simulink model "Analisis_de_Ganancias"  (R2023a)
settings: Solver=VariableStepAuto  StartTime=0.0  StopTime=10.0  RelTol=1e-3
undefined symbols (not defined in the file): alfa_inicial, area_mem, c, d, delta_f, fs, k, m, perm, Q, r1, r_ambiente1, r_ambiente2, rho, v_sonido, vel_caminata, ventana_fft, ventana_fft_analisis, zoh_freq
libraries: matrix_library x4, dspxfrm3 x2, dspvision x2, dspsnks4 x1
settings Model: Creator=tobip  LastModifiedBy=tobip

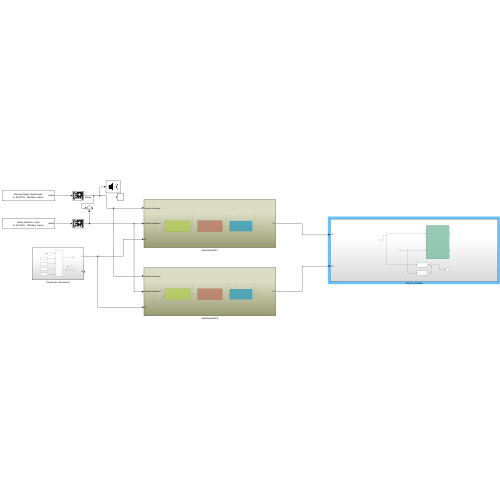
[thumbnail: Simulink's stored preview of the top-level diagram]
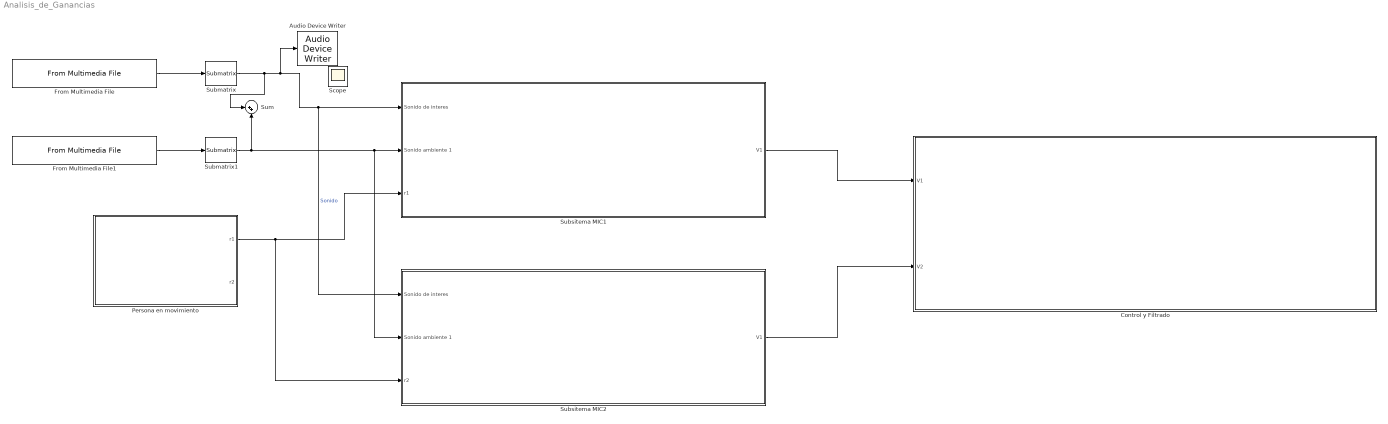
== system Analisis_de_Ganancias ==
  Audio Device Writer : dspsnks4/Audio Device Writer  Driver=DirectSound  Device=Default  InheritSampleRate=on  SampleRate=44100  BitDepth=16-bit integer  BufferSize=4096  NumBuffers=10  DefaultOutputChannelMapping=on  OutputChannelMapping=1:2  OutputNumUnderrunSamples=off  DriverIdx=1  DeviceWarnFlag=''
  Control y Filtrado : Subsystem
  From Multimedia File : dspvision/From Multimedia File  inputFilename=C:\Users\tobip\Documents\Control\Proyecto final\Audios dato\Discurso Roger Federer.mp3  readRange=[1 Inf]  loop=on  numPlays=1  outputStreams=Audio only  videoDataType=single  audioDataType=double  inheritSampleTime=on  userDefinedSampleTime=1/30  noAudioOutput=off  isIntensityVideo=off  fourcc=RGB  colorVideoFormat=Separate color signals  outputEOF=off  dataOrg=Column-major  audioFrameSize=1  computeAudioFrameSize=off  outSamplingMode=Sample based
      settings: LibrarySourceBlock=audiosources/From Multimedia File
  From Multimedia File1 : dspvision/From Multimedia File  inputFilename=C:\Users\tobip\Documents\Control\Proyecto final\Audios dato\Ruido ambiente 1.mp3  readRange=[1 Inf]  loop=on  numPlays=1  outputStreams=Audio only  videoDataType=single  audioDataType=double  inheritSampleTime=on  userDefinedSampleTime=1/30  noAudioOutput=off  isIntensityVideo=off  fourcc=RGB  colorVideoFormat=Separate color signals  outputEOF=off  dataOrg=Column-major  audioFrameSize=1  computeAudioFrameSize=off  outSamplingMode=Sample based
      settings: LibrarySourceBlock=audiosources/From Multimedia File
  Persona en movimiento : Subsystem
  Scope : Scope
  Submatrix : matrix_library/Submatrix  RowSpan=All rows  RowStartMode=First  RowStartIndex=1  RowEndMode=Middle  RowEndIndex=1  ColSpan=One column  ColStartMode=First  ColStartIndex=1  ColEndMode=Last  ColEndIndex=1
  Submatrix1 : matrix_library/Submatrix  RowSpan=All rows  RowStartMode=First  RowStartIndex=1  RowEndMode=Last  RowEndIndex=1  ColSpan=One column  ColStartMode=First  ColStartIndex=1  ColEndMode=Last  ColEndIndex=1
  Subsitema MIC1 : Subsystem
  Subsitema MIC2 : Subsystem
  Sum : Sum  Inputs=|++
  wires:
  Subsitema MIC2/1(V1) -> Control y Filtrado/2(V2)
  Persona en movimiento/1(r1) -> Subsitema MIC2/3(r2), Subsitema MIC1/3(r1)
  Submatrix1/1 -> Subsitema MIC2/2(Sonido ambiente 1), Subsitema MIC1/2(Sonido ambiente 1), Sum/2
  Submatrix/1 -> Sum/1, Audio Device Writer/1, Subsitema MIC1/1(Sonido de interes), Subsitema MIC2/1(Sonido de interes)  "Sonido"
  Subsitema MIC1/1(V1) -> Control y Filtrado/1(V1)
  From Multimedia File1/1 -> Submatrix1/1
  From Multimedia File/1 -> Submatrix/1

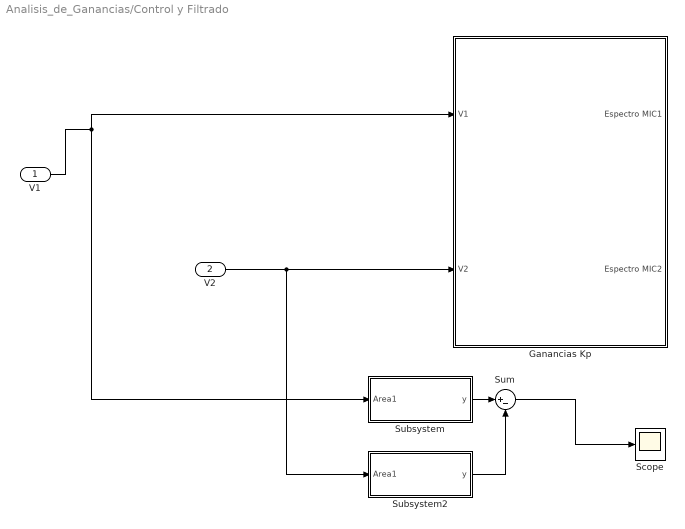
== system Analisis_de_Ganancias/Control y Filtrado ==
  V1 : Inport
  V2 : Inport  Port=2
  Ganancias Kp : Subsystem
  Scope : Scope
  Subsystem : Subsystem
  Subsystem2 : Subsystem
  Sum : Sum  Inputs=|+-
  wires:
  Subsystem/1(y) -> Sum/1
  Subsystem2/1(y) -> Sum/2
  Sum/1 -> Scope/1
  V1/1 -> Ganancias Kp/1(V1), Subsystem/1(Area1)
  V2/1 -> Ganancias Kp/2(V2), Subsystem2/1(Area1)

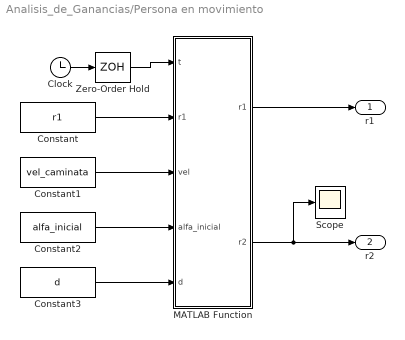
== system Analisis_de_Ganancias/Persona en movimiento ==
  Clock : Clock
  Constant : Constant  Value=r1
  Constant1 : Constant  Value=vel_caminata
  Constant2 : Constant  Value=alfa_inicial
  Constant3 : Constant  Value=d
  MATLAB Function : MATLAB Function  TreatAsAtomicUnit=on
  Scope : Scope
  Zero-Order Hold : ZeroOrderHold  SampleTime=0.1
  r1 : Outport
  r2 : Outport  Port=2
  wires:
  Constant/1 -> MATLAB Function/2("r1 ")
  Constant3/1 -> MATLAB Function/5(d)
  Constant2/1 -> MATLAB Function/4(alfa_inicial)
  Constant1/1 -> MATLAB Function/3(vel)
  Clock/1 -> Zero-Order Hold/1
  MATLAB Function/1(r1) -> r1/1
  Zero-Order Hold/1 -> MATLAB Function/1(t)
  MATLAB Function/2(r2) -> Scope/1, r2/1

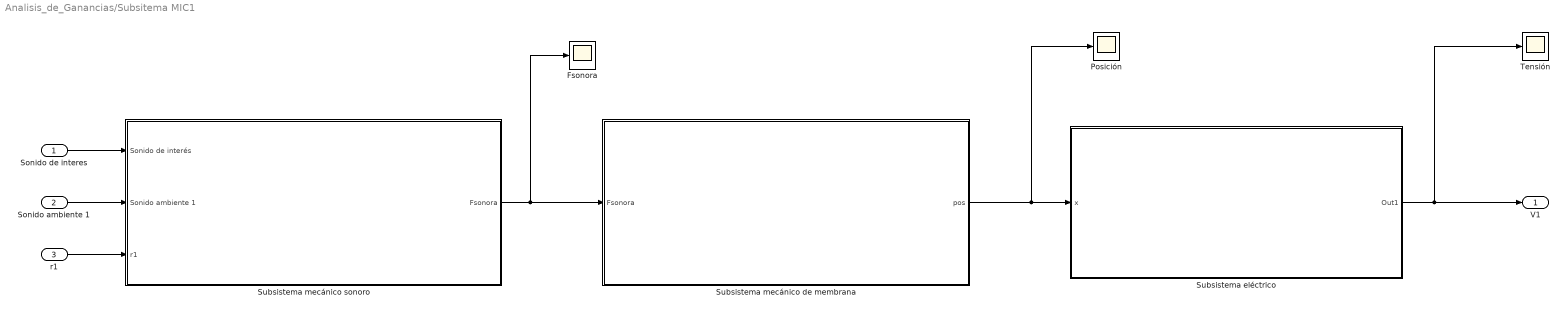
== system Analisis_de_Ganancias/Subsitema MIC1 ==
  Sonido de interes : Inport
  Sonido ambiente 1 : Inport  Port=2
  r1 : Inport  Port=3
  Fsonora : Scope
  Posición : Scope
  Subsistema eléctrico : Subsystem
  Subsistema mecánico de membrana : Subsystem
  Subsistema mecánico sonoro : Subsystem
  Tensión : Scope
  V1 : Outport
  wires:
  Subsistema mecánico de membrana/1(pos) -> Posición/1, Subsistema eléctrico/1(x)
  Sonido de interes/1 -> Subsistema mecánico sonoro/1(Sonido de interés)
  Subsistema eléctrico/1(Out1) -> Tensión/1, V1/1
  Subsistema mecánico sonoro/1(Fsonora) -> Fsonora/1, Subsistema mecánico de membrana/1(Fsonora)
  Sonido ambiente 1/1 -> Subsistema mecánico sonoro/2(Sonido ambiente 1)
  r1/1 -> Subsistema mecánico sonoro/3(r1)

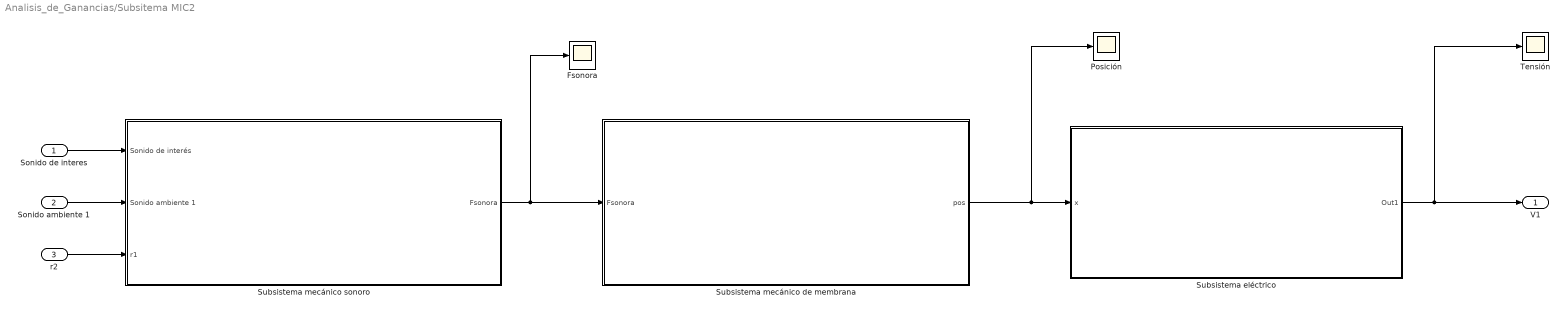
== system Analisis_de_Ganancias/Subsitema MIC2 ==
  Sonido de interes : Inport
  Sonido ambiente 1 : Inport  Port=2
  r2 : Inport  Port=3
  Fsonora : Scope
  Posición : Scope
  Subsistema eléctrico : Subsystem
  Subsistema mecánico de membrana : Subsystem
  Subsistema mecánico sonoro : Subsystem
  Tensión : Scope
  V1 : Outport
  wires:
  Subsistema mecánico de membrana/1(pos) -> Posición/1, Subsistema eléctrico/1(x)
  Sonido de interes/1 -> Subsistema mecánico sonoro/1(Sonido de interés)
  Subsistema eléctrico/1(Out1) -> Tensión/1, V1/1
  Subsistema mecánico sonoro/1(Fsonora) -> Fsonora/1, Subsistema mecánico de membrana/1(Fsonora)
  Sonido ambiente 1/1 -> Subsistema mecánico sonoro/2(Sonido ambiente 1)
  r2/1 -> Subsistema mecánico sonoro/3(r1)

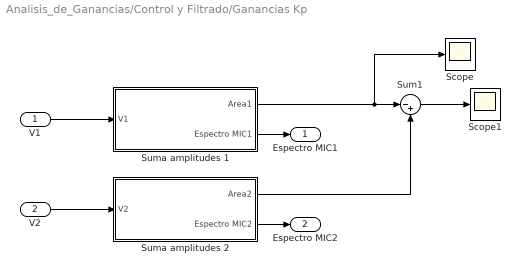
== system Analisis_de_Ganancias/Control y Filtrado/Ganancias Kp ==
  V1 : Inport
  V2 : Inport  Port=2
  Scope : Scope
  Scope1 : Scope
  Sum1 : Sum  Inputs=|-+
  Suma amplitudes 1 : Subsystem
  Suma amplitudes 2 : Subsystem
  Espectro MIC1 : Outport
  Espectro MIC2 : Outport  Port=2
  wires:
  V1/1 -> Suma amplitudes 1/1(V1)
  V2/1 -> Suma amplitudes 2/1(V2)
  Suma amplitudes 1/2(Espectro MIC1) -> Espectro MIC1/1
  Suma amplitudes 2/2(Espectro MIC2) -> Espectro MIC2/1
  Suma amplitudes 1/1(Area1) -> Scope/1, Sum1/1
  Sum1/1 -> Scope1/1
  Suma amplitudes 2/1(Area2) -> Sum1/2

== system Analisis_de_Ganancias/Control y Filtrado/Subsystem ==
  Area1 : Inport
  Buffer : Buffer  N=3  OutputFrames=off
  MATLAB Function : MATLAB Function  TreatAsAtomicUnit=on
  Zero-Order Hold : ZeroOrderHold  SampleTime=1/fs
  y : Outport
  wires:
  Buffer/1 -> MATLAB Function/1(u)
  Area1/1 -> Zero-Order Hold/1
  MATLAB Function/1(y) -> y/1
  Zero-Order Hold/1 -> Buffer/1

== system Analisis_de_Ganancias/Control y Filtrado/Subsystem2 ==
  Area1 : Inport
  Buffer : Buffer  N=3  OutputFrames=off
  MATLAB Function : MATLAB Function  TreatAsAtomicUnit=on
  Zero-Order Hold : ZeroOrderHold  SampleTime=1/fs
  y : Outport
  wires:
  Buffer/1 -> MATLAB Function/1(u)
  Area1/1 -> Zero-Order Hold/1
  MATLAB Function/1(y) -> y/1
  Zero-Order Hold/1 -> Buffer/1

== system Analisis_de_Ganancias/Subsitema MIC1/Subsistema eléctrico ==
  x : Inport
  Constant : Constant  Value=area_mem*perm
  Constant1 : Constant  Value=Q
  Divide : Product  Inputs=*/
  Divide1 : Product  Inputs=*/
  Out1 : Outport
  wires:
  x/1 -> Divide/2
  Constant/1 -> Divide/1
  Divide/1 -> Divide1/2  "Capacitancia"
  Divide1/1 -> Out1/1
  Constant1/1 -> Divide1/1

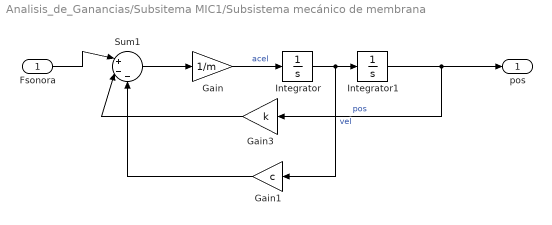
== system Analisis_de_Ganancias/Subsitema MIC1/Subsistema mecánico de membrana ==
  Fsonora : Inport
  Gain : Gain  Gain=1/m
  Gain1 : Gain  Gain=c
  Gain3 : Gain  Gain=k
  Integrator : Integrator
  Integrator1 : Integrator
  Sum1 : Sum  Inputs=|+--
  pos : Outport
  wires:
  Integrator1/1 -> Gain3/1, pos/1  "pos"
  Integrator/1 -> Gain1/1, Integrator1/1  "vel"
  Fsonora/1 -> Sum1/1
  Gain3/1 -> Sum1/2
  Sum1/1 -> Gain/1
  Gain/1 -> Integrator/1  "acel"
  Gain1/1 -> Sum1/3

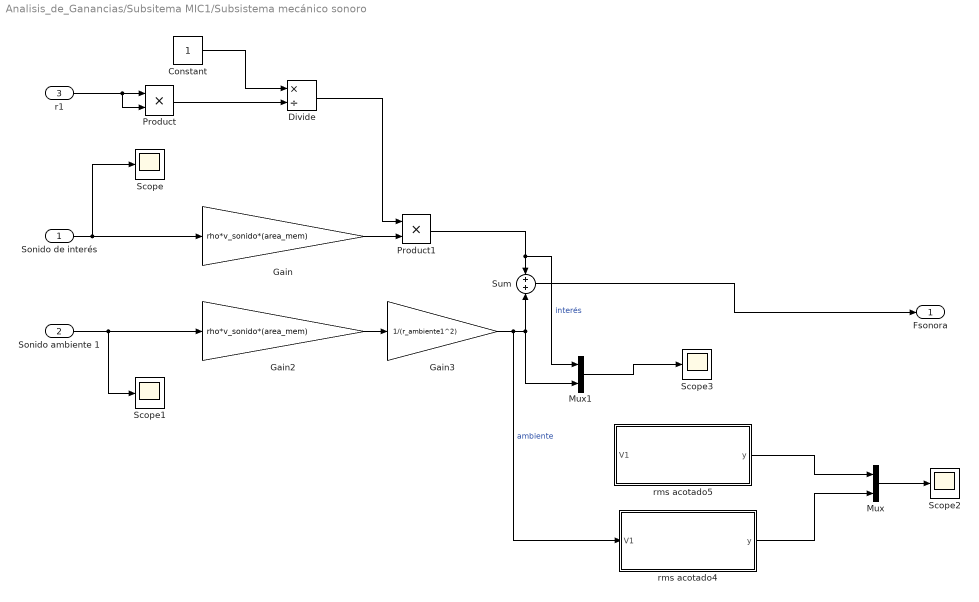
== system Analisis_de_Ganancias/Subsitema MIC1/Subsistema mecánico sonoro ==
  Sonido de interés : Inport
  Sonido ambiente 1 : Inport  Port=2
  r1 : Inport  Port=3
  Constant : Constant
  Divide : Product  Inputs=*/
  Gain : Gain  Gain=rho*v_sonido*(area_mem)
  Gain2 : Gain  Gain=rho*v_sonido*(area_mem)
  Gain3 : Gain  Gain=1/(r_ambiente1^2)
  Mux : Mux  Inputs=2
  Mux1 : Mux  Inputs=2
  Product : Product
  Product1 : Product
  Scope{,1..3} (4 alike) : Scope
  Sum : Sum
  rms acotado4 : Subsystem
  rms acotado5 : Subsystem
  Fsonora : Outport
  wires:
  Gain/1 -> Product1/2
  Sonido de interés/1 -> Gain/1, Scope/1
  Gain2/1 -> Gain3/1
  Gain3/1 -> rms acotado4/1(V1), Sum/2, Mux1/2  "ambiente"
  Sonido ambiente 1/1 -> Scope1/1, Gain2/1
  rms acotado5/1(y) -> Mux/1
  rms acotado4/1(y) -> Mux/2
  Mux/1 -> Scope2/1
  r1/1 -> Product/2, Product/1
  Product/1 -> Divide/2
  Constant/1 -> Divide/1
  Divide/1 -> Product1/1
  Product1/1 -> Mux1/1, Sum/1  "interés"
  Mux1/1 -> Scope3/1
  Sum/1 -> Fsonora/1

== system Analisis_de_Ganancias/Subsitema MIC2/Subsistema eléctrico ==
  x : Inport
  Constant : Constant  Value=area_mem*perm
  Constant1 : Constant  Value=Q
  Divide : Product  Inputs=*/
  Divide1 : Product  Inputs=*/
  Out1 : Outport
  wires:
  x/1 -> Divide/2
  Constant/1 -> Divide/1
  Divide/1 -> Divide1/2  "Capacitancia"
  Divide1/1 -> Out1/1
  Constant1/1 -> Divide1/1

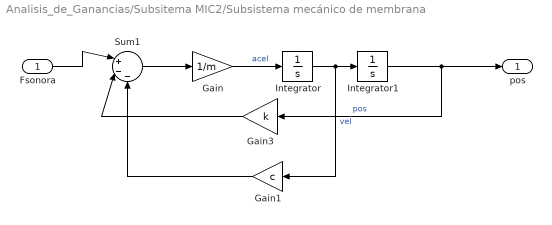
== system Analisis_de_Ganancias/Subsitema MIC2/Subsistema mecánico de membrana ==
  Fsonora : Inport
  Gain : Gain  Gain=1/m
  Gain1 : Gain  Gain=c
  Gain3 : Gain  Gain=k
  Integrator : Integrator
  Integrator1 : Integrator
  Sum1 : Sum  Inputs=|+--
  pos : Outport
  wires:
  Integrator1/1 -> Gain3/1, pos/1  "pos"
  Integrator/1 -> Gain1/1, Integrator1/1  "vel"
  Fsonora/1 -> Sum1/1
  Gain3/1 -> Sum1/2
  Sum1/1 -> Gain/1
  Gain/1 -> Integrator/1  "acel"
  Gain1/1 -> Sum1/3

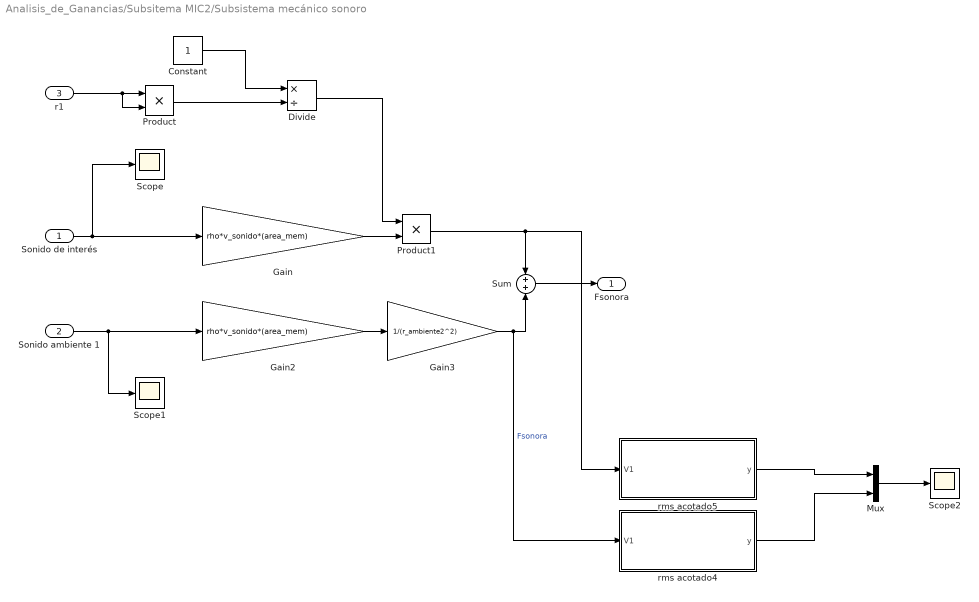
== system Analisis_de_Ganancias/Subsitema MIC2/Subsistema mecánico sonoro ==
  Sonido de interés : Inport
  Sonido ambiente 1 : Inport  Port=2
  r1 : Inport  Port=3
  Constant : Constant
  Divide : Product  Inputs=*/
  Gain : Gain  Gain=rho*v_sonido*(area_mem)
  Gain2 : Gain  Gain=rho*v_sonido*(area_mem)
  Gain3 : Gain  Gain=1/(r_ambiente2^2)
  Mux : Mux  Inputs=2
  Product : Product
  Product1 : Product
  Scope : Scope
  Scope1 : Scope
  Scope2 : Scope
  Sum : Sum
  rms acotado4 : Subsystem
  rms acotado5 : Subsystem
  Fsonora : Outport
  wires:
  Gain/1 -> Product1/2
  Sonido de interés/1 -> Gain/1, Scope/1
  Gain2/1 -> Gain3/1
  Gain3/1 -> rms acotado4/1(V1), Sum/2  "Fsonora"
  Sonido ambiente 1/1 -> Scope1/1, Gain2/1
  rms acotado5/1(y) -> Mux/1
  rms acotado4/1(y) -> Mux/2
  Mux/1 -> Scope2/1
  r1/1 -> Product/2, Product/1
  Product/1 -> Divide/2
  Constant/1 -> Divide/1
  Divide/1 -> Product1/1
  Product1/1 -> rms acotado5/1(V1), Sum/1
  Sum/1 -> Fsonora/1

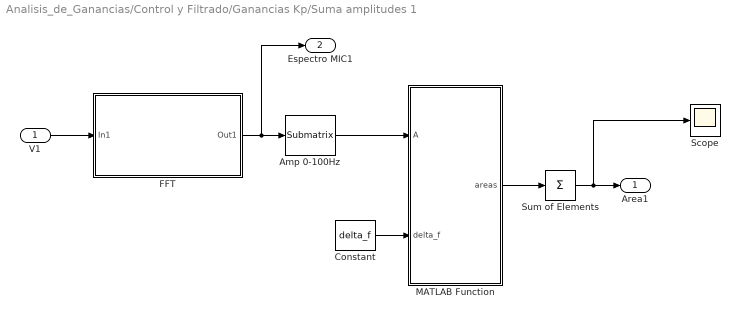
== system Analisis_de_Ganancias/Control y Filtrado/Ganancias Kp/Suma amplitudes 1 ==
  V1 : Inport
  Amp 0-100Hz : matrix_library/Submatrix  RowSpan=Range of rows  RowStartMode=Index  RowStartIndex=20  RowEndMode=Index  RowEndIndex=160  ColSpan=One column  ColStartMode=First  ColStartIndex=1  ColEndMode=Last  ColEndIndex=1
  Constant : Constant  Value=delta_f
  FFT : Subsystem
  MATLAB Function : MATLAB Function  TreatAsAtomicUnit=on
  Scope : Scope
  Sum of Elements : Sum  Inputs=+
  Area1 : Outport
  Espectro MIC1 : Outport  Port=2
  wires:
  Amp 0-100Hz/1 -> MATLAB Function/1(A)
  Constant/1 -> MATLAB Function/2(delta_f)
  MATLAB Function/1(areas) -> Sum of Elements/1
  Sum of Elements/1 -> Scope/1, Area1/1
  FFT/1(Out1) -> Espectro MIC1/1, Amp 0-100Hz/1
  V1/1 -> FFT/1(In1)

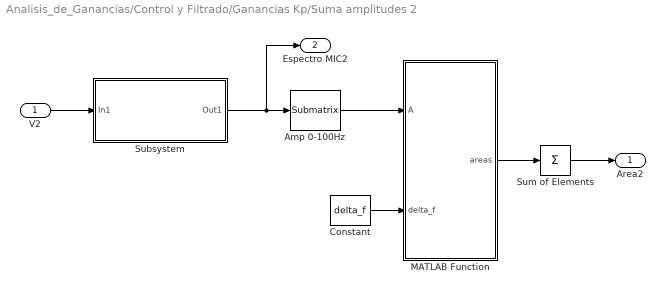
== system Analisis_de_Ganancias/Control y Filtrado/Ganancias Kp/Suma amplitudes 2 ==
  V2 : Inport
  Amp 0-100Hz : matrix_library/Submatrix  RowSpan=Range of rows  RowStartMode=Index  RowStartIndex=20  RowEndMode=Index  RowEndIndex=160  ColSpan=One column  ColStartMode=First  ColStartIndex=1  ColEndMode=Last  ColEndIndex=1
  Constant : Constant  Value=delta_f
  MATLAB Function : MATLAB Function  TreatAsAtomicUnit=on
  Subsystem : Subsystem
  Sum of Elements : Sum  Inputs=+
  Area2 : Outport
  Espectro MIC2 : Outport  Port=2
  wires:
  Amp 0-100Hz/1 -> MATLAB Function/1(A)
  Constant/1 -> MATLAB Function/2(delta_f)
  MATLAB Function/1(areas) -> Sum of Elements/1
  Sum of Elements/1 -> Area2/1
  Subsystem/1(Out1) -> Espectro MIC2/1, Amp 0-100Hz/1
  V2/1 -> Subsystem/1(In1)

== system Analisis_de_Ganancias/Subsitema MIC1/Subsistema mecánico sonoro/rms acotado4 ==
  V1 : Inport
  Buffer : Buffer  N=20  OutputFrames=off
  MATLAB Function : MATLAB Function  TreatAsAtomicUnit=on
  Zero-Order Hold : ZeroOrderHold  SampleTime=zoh_freq
  y : Outport
  wires:
  MATLAB Function/1(y) -> y/1
  Buffer/1 -> MATLAB Function/1(u)
  V1/1 -> Zero-Order Hold/1
  Zero-Order Hold/1 -> Buffer/1

== system Analisis_de_Ganancias/Subsitema MIC1/Subsistema mecánico sonoro/rms acotado5 ==
  V1 : Inport
  Buffer : Buffer  N=20  OutputFrames=off
  MATLAB Function : MATLAB Function  TreatAsAtomicUnit=on
  Zero-Order Hold : ZeroOrderHold  SampleTime=zoh_freq
  y : Outport
  wires:
  MATLAB Function/1(y) -> y/1
  Buffer/1 -> MATLAB Function/1(u)
  V1/1 -> Zero-Order Hold/1
  Zero-Order Hold/1 -> Buffer/1

== system Analisis_de_Ganancias/Subsitema MIC2/Subsistema mecánico sonoro/rms acotado4 ==
  V1 : Inport
  Buffer : Buffer  N=20  OutputFrames=off
  MATLAB Function : MATLAB Function  TreatAsAtomicUnit=on
  Zero-Order Hold : ZeroOrderHold  SampleTime=zoh_freq
  y : Outport
  wires:
  MATLAB Function/1(y) -> y/1
  Buffer/1 -> MATLAB Function/1(u)
  V1/1 -> Zero-Order Hold/1
  Zero-Order Hold/1 -> Buffer/1

== system Analisis_de_Ganancias/Subsitema MIC2/Subsistema mecánico sonoro/rms acotado5 ==
  V1 : Inport
  Buffer : Buffer  N=20  OutputFrames=off
  MATLAB Function : MATLAB Function  TreatAsAtomicUnit=on
  Zero-Order Hold : ZeroOrderHold  SampleTime=zoh_freq
  y : Outport
  wires:
  MATLAB Function/1(y) -> y/1
  Buffer/1 -> MATLAB Function/1(u)
  V1/1 -> Zero-Order Hold/1
  Zero-Order Hold/1 -> Buffer/1

== system Analisis_de_Ganancias/Control y Filtrado/Ganancias Kp/Suma amplitudes 1/FFT ==
  In1 : Inport
  Buffer : Buffer  N=ventana_fft  V=ventana_fft_analisis-1  OutputFrames=off
  Complex to Magnitude-Angle : ComplexToMagnitudeAngle  Output=Magnitude
  FFT : dspxfrm3/FFT  FFTImplementation=Auto  CompMethod=Table lookup  TableOpt=NEW  TableOptActive=Speed  BitRevOrder=off  Normalize=off  InheritFFTLength=on  FFTLength=64  WrapInput=on  roundingMode=Floor  overflowMode=off  firstCoeffDataTypeStr=Inherit: Same word length as input  firstCoeffLastDataTypeStr=Inherit: Same word length as input  outputMin=[]  outputMax=[]
  Zero-Order Hold : ZeroOrderHold  SampleTime=zoh_freq
  Out1 : Outport
  wires:
  Complex to Magnitude-Angle/1 -> Out1/1
  FFT/1 -> Complex to Magnitude-Angle/1
  In1/1 -> Zero-Order Hold/1
  Buffer/1 -> FFT/1
  Zero-Order Hold/1 -> Buffer/1

== system Analisis_de_Ganancias/Control y Filtrado/Ganancias Kp/Suma amplitudes 2/Subsystem ==
  In1 : Inport
  Buffer : Buffer  N=ventana_fft  V=ventana_fft_analisis-1  OutputFrames=off
  Complex to Magnitude-Angle : ComplexToMagnitudeAngle  Output=Magnitude
  FFT : dspxfrm3/FFT  FFTImplementation=Auto  CompMethod=Table lookup  TableOpt=NEW  TableOptActive=Speed  BitRevOrder=off  Normalize=off  InheritFFTLength=on  FFTLength=64  WrapInput=on  roundingMode=Floor  overflowMode=off  firstCoeffDataTypeStr=Inherit: Same word length as input  firstCoeffLastDataTypeStr=Inherit: Same word length as input  outputMin=[]  outputMax=[]
  Zero-Order Hold : ZeroOrderHold  SampleTime=zoh_freq
  Out1 : Outport
  wires:
  In1/1 -> Zero-Order Hold/1
  Complex to Magnitude-Angle/1 -> Out1/1
  FFT/1 -> Complex to Magnitude-Angle/1
  Buffer/1 -> FFT/1
  Zero-Order Hold/1 -> Buffer/1

== matlab function Analisis_de_Ganancias/Control y Filtrado/Ganancias Kp/Suma amplitudes 2/MATLAB Function ==
  data: A input; areas output; delta_f input
function areas = fcn(A, delta_f)

areas = A.* delta_f;

== matlab function Analisis_de_Ganancias/Control y Filtrado/Ganancias Kp/Suma amplitudes 1/MATLAB Function ==
  data: A input; areas output; delta_f input
function areas = fcn(A, delta_f)

areas = A.* delta_f;

== matlab function Analisis_de_Ganancias/Subsitema MIC2/Subsistema mecánico sonoro/rms acotado4/MATLAB Function ==
  data: u input; y output
function y = fcn(u)
% y=0;
%     for i=1:length(u)
%         y = y + u(i)^2;
%     end
%     y=sqrt(y);
    y = sqrt(mean(u.^2));

== matlab function Analisis_de_Ganancias/Persona en movimiento/MATLAB Function ==
  settings: updateMethod=DISCRETE
  data: t input; r1 output; r1 input; vel input; alfa_inicial input; d input; r2 output
function [r1, r2] = fcn(t, r1, vel, alfa_inicial, d)

% persistent h fig

omega = vel/r1;
alfa = alfa_inicial + omega*t;
r2 = sqrt((r1^2) + (d^2) - 2*r1*d*cos(alfa));   %Distancia a mic2

x1 = r1*cos(alfa);
y1 = r1*sin(alfa);

% % Inicializar el gráfico
% if isempty(h)
%     fig = figure('Name', 'Caminata en el plano', 'NumberTitle', 'off');
%     h = plot(0, 0, 'ro', 'MarkerSize', 10, 'MarkerFaceColor', 'r');
%     axis([-1 1 -1 1]); % Ajusta los límites según el rango de tu simulación
%     grid on;
%     xlabel('X (m)');
%     ylabel('Y (m)');
%     title('Caminata en el plano');
% end
% 
% % Actualizar el punto
% if ishandle(h)  % Cambiado de 'isvalid' a 'ishandle'
%     set(h, 'XData', x1, 'YData', y1);
%     hold on
%      plot(d/2, 0, 'ro' ,'MarkerSize', 30, 'MarkerFaceColor', 'k');
%     plot(0, 0, 'ro' ,'MarkerSize', 4, 'MarkerFaceColor', 'b');
%     plot(d, 0, 'ro' ,'MarkerSize', 4, 'MarkerFaceColor', 'b');
%     hold off
%     drawnow;
% end
end

== matlab function Analisis_de_Ganancias/Subsitema MIC2/Subsistema mecánico sonoro/rms acotado5/MATLAB Function ==
  data: u input; y output
function y = fcn(u)
% y=0;
%     for i=1:length(u)
%         y = y + u(i)^2;
%     end
%     y=sqrt(y);
    y = sqrt(mean(u.^2));

== matlab function Analisis_de_Ganancias/Subsitema MIC1/Subsistema mecánico sonoro/rms acotado4/MATLAB Function ==
  data: u input; y output
function y = fcn(u)
% y=0;
%     for i=1:length(u)
%         y = y + u(i)^2;
%     end
%     y=sqrt(y);
    y = sqrt(mean(u.^2));

== matlab function Analisis_de_Ganancias/Subsitema MIC1/Subsistema mecánico sonoro/rms acotado5/MATLAB Function ==
  data: u input; y output
function y = fcn(u)
% y=0;
%     for i=1:length(u)
%         y = y + u(i)^2;
%     end
%     y=sqrt(y);
    y = sqrt(mean(u.^2));

== matlab function Analisis_de_Ganancias/Control y Filtrado/Subsystem/MATLAB Function ==
  data: u input; y output
function y = square_elements(u)
    y = sqrt(mean(u.^2));

== matlab function Analisis_de_Ganancias/Control y Filtrado/Subsystem2/MATLAB Function ==
  data: u input; y output
function y = square_elements(u)
    y = sqrt(mean(u.^2));
